simulink library "env2turbLinearize_cl"  (R2020a)
settings: Solver=VariableStepAuto  StartTime=0.0  StopTime=10.0  RelTol=1e-3
undefined symbols (not defined in the file or in its folder): distAmp, distFreq, flwSpd, initializeBussesFromBlock, pertVec, vhcl
libraries: flowcalculation_cl x4, $bdroot x3, eulAng2RotMat_ul x1, alphaBetaLE_ul x1, vrlib x1
settings Model: Creator=mcobb  LastModifiedBy=andre
settings DataIOCC: ReturnWorkspaceOutputs=off
settings DebuggingCC: ArithmeticOperatorsInVariantConditions=warning
settings SFSimCC: CustomCodeUndefinedFunction=UseInterfaceOnly

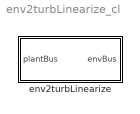
== system env2turbLinearize_cl ==
  env2turbLinearize : Subsystem  LoadFcn=initializeBussesFromBlock(gcb)  InitFcn=initializeBussesFromBlock(gcb)  StartFcn=initializeBussesFromBlock(gcb)
      settings: MinAlgLoopOccurrences=on

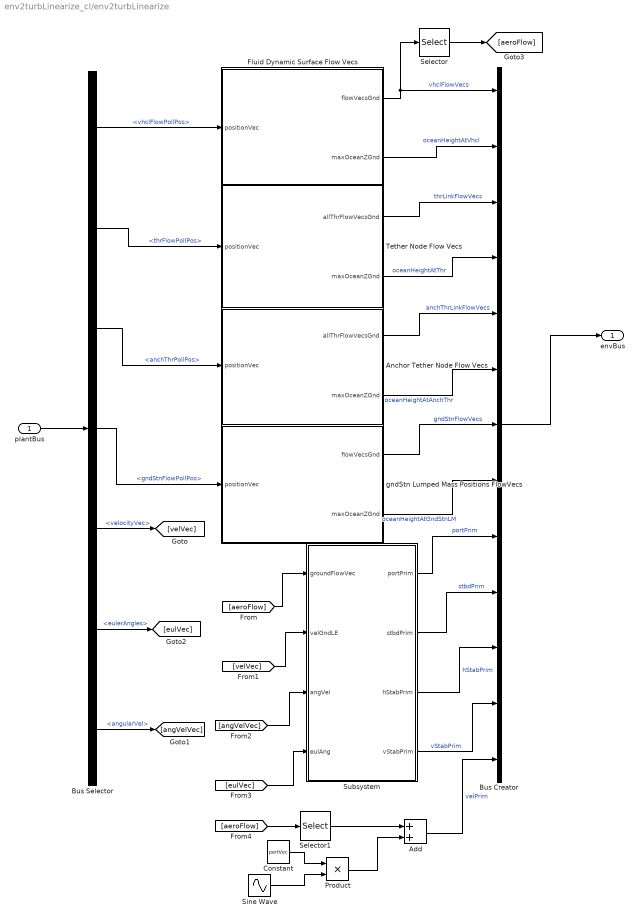
== system env2turbLinearize_cl/env2turbLinearize ==
  plantBus : Inport  OutDataTypeStr=Bus: plantBus
  Add : Sum
  Anchor Tether Node Flow Vecs : Subsystem
  Bus Creator : BusCreator  Inputs=13  OutDataTypeStr=Bus: envBus  NonVirtualBus=on
  Bus Selector : BusSelector  OutputSignals=vhclFlowPollPos,thrFlowPollPos,anchThrPollPos,gndStnFlowPollPos,velocityVec,eulerAngles,angularVel
  Constant : Constant  Value=pertVec
  Fluid Dynamic Surface Flow Vecs : Subsystem
      settings: MinAlgLoopOccurrences=on
  Product : Product
  Selector : Selector  NumberOfDimensions=2  InputPortWidth=[13 3]  IndexOptions=Select all,Index vector (dialog)  Indices=[1 3],[1 2 3 4]  OutputSizes=1,1
  Selector1 : Selector  NumberOfDimensions=2  InputPortWidth=3  IndexOptions=Select all,Index vector (dialog)  Indices=[1 3],1  OutputSizes=1,1
  Sine Wave : Sin  Amplitude=distAmp*flwSpd  Frequency=distFreq*2*pi  SampleTime=[0,1]
  Subsystem : Subsystem  mask{vhcl=vhcl, fluidMomentArms=vhcl.fluidMomentArms.Value}
      mask prompts: vhcl "Vehicle Object"; fluidMomentArms "Fluid Moment Arms"
  Tether Node Flow Vecs : Subsystem
      settings: MinAlgLoopOccurrences=on
  gndStn Lumped Mass Positions FlowVecs : Subsystem
      settings: MinAlgLoopOccurrences=on
  envBus : Outport  OutDataTypeStr=Bus: envBus  VectorParamsAs1DForOutWhenUnconnected=off
  wires:
  Bus Selector/1 -> Fluid Dynamic Surface Flow Vecs/1(positionVec)  "<vhclFlowPollPos>"
  Fluid Dynamic Surface Flow Vecs/1(flowVecsGnd) -> Selector/1, Bus Creator/1  "vhclFlowVecs"
  Bus Creator/1 -> envBus/1
  Bus Selector/3 -> Anchor Tether Node Flow Vecs/1(positionVec)  "<anchThrPollPos>"
  Bus Selector/2 -> Tether Node Flow Vecs/1(positionVec)  "<thrFlowPollPos>"
  plantBus/1 -> Bus Selector/1
  Bus Selector/4 -> gndStn Lumped Mass Positions FlowVecs/1(positionVec)  "<gndStnFlowPollPos>"
  gndStn Lumped Mass Positions FlowVecs/2(maxOceanZGnd) -> Bus Creator/8  "oceanHeightAtGndStnLM"
  Tether Node Flow Vecs/1(allThrFlowVecsGnd) -> Bus Creator/3  "thrLinkFlowVecs"
  Anchor Tether Node Flow Vecs/1(allThrFlowVecsGnd) -> Bus Creator/5  "anchThrLinkFlowVecs"
  gndStn Lumped Mass Positions FlowVecs/1(flowVecsGnd) -> Bus Creator/7  "gndStnFlowVecs"
  Anchor Tether Node Flow Vecs/2(maxOceanZGnd) -> Bus Creator/6  "oceanHeightAtAnchThr"
  Tether Node Flow Vecs/2(maxOceanZGnd) -> Bus Creator/4  "oceanHeightAtThr"
  Fluid Dynamic Surface Flow Vecs/2(maxOceanZGnd) -> Bus Creator/2  "oceanHeightAtVhcl"
  Bus Selector/5 -> [velVec]  "<velocityVec>"
  Bus Selector/7 -> [angVelVec]  "<angularVel>"
  Bus Selector/6 -> [eulVec]  "<eulerAngles>"
  [velVec] -> Subsystem/2(velGndLE)
  Selector/1 -> [aeroFlow]
  [aeroFlow] -> Subsystem/1(groundFlowVec)
  [angVelVec] -> Subsystem/3(angVel)
  [eulVec] -> Subsystem/4(eulAng)
  Subsystem/2(stbdPrim) -> Bus Creator/10  "stbdPrim"
  Subsystem/3(hStabPrim) -> Bus Creator/11  "hStabPrim"
  Subsystem/4(vStabPrim) -> Bus Creator/12  "vStabPrim"
  Subsystem/1(portPrim) -> Bus Creator/9  "portPrim"
  [aeroFlow] -> Selector1/1
  Selector1/1 -> Add/1
  Sine Wave/1 -> Product/2
  Add/1 -> Bus Creator/13  "velPrim"
  Constant/1 -> Product/1
  Product/1 -> Add/2

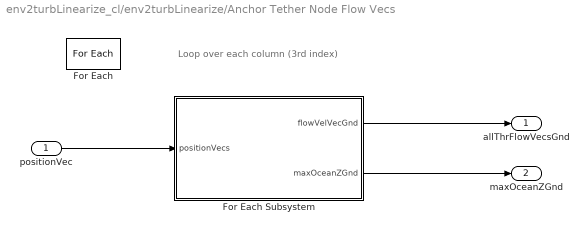
== system env2turbLinearize_cl/env2turbLinearize/Anchor Tether Node Flow Vecs ==
  note: Loop over each column (3rd index)
  positionVec : Inport  Partition=on  PartitionDimension=3  PartitionWidth=1  PartitionOffset=0
  For Each : ForEach  DisableCoverage=on
  For Each Subsystem : Subsystem
      settings: MinAlgLoopOccurrences=on
  allThrFlowVecsGnd : Outport  ConcatenationDimension=3  VectorParamsAs1DForOutWhenUnconnected=off
  maxOceanZGnd : Outport  Port=2  ConcatenationDimension=1  VectorParamsAs1DForOutWhenUnconnected=off
  wires:
  positionVec/1 -> For Each Subsystem/1(positionVecs)
  For Each Subsystem/1(flowVelVecGnd) -> allThrFlowVecsGnd/1
  For Each Subsystem/2(maxOceanZGnd) -> maxOceanZGnd/1

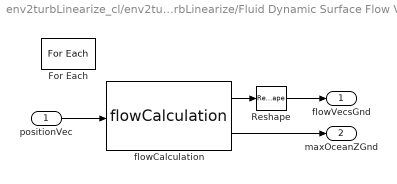
== system env2turbLinearize_cl/env2turbLinearize/Fluid Dynamic Surface Flow Vecs ==
  positionVec : Inport  Partition=on  PartitionDimension=2  PartitionWidth=1  PartitionOffset=0
  For Each : ForEach  DisableCoverage=on
  Reshape : Reshape  OutputDimensionality=Column vector (2-D)
  flowCalculation : flowcalculation_cl/flowCalculation  SystemSampleTime=-1  Latency=0  AutoFrameSizeCalculation=off
  flowVecsGnd : Outport  ConcatenationDimension=2  VectorParamsAs1DForOutWhenUnconnected=off
  maxOceanZGnd : Outport  Port=2  ConcatenationDimension=1  VectorParamsAs1DForOutWhenUnconnected=off
  wires:
  positionVec/1 -> flowCalculation/1
  flowCalculation/1 -> Reshape/1
  Reshape/1 -> flowVecsGnd/1
  flowCalculation/2 -> maxOceanZGnd/1

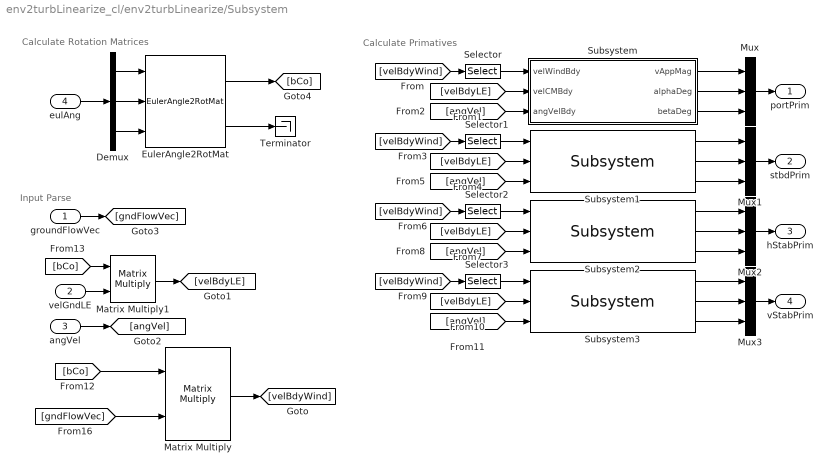
== system env2turbLinearize_cl/env2turbLinearize/Subsystem ==
  note: Calculate Primatives
  note: Calculate Rotation Matrices
  note: Input Parse
  groundFlowVec : Inport
  velGndLE : Inport  Port=2
  angVel : Inport  Port=3
  eulAng : Inport  Port=4
  Demux : Demux  Outputs=3
  EulerAngle2RotMat : eulAng2RotMat_ul/EulerAngle2RotMat  SystemSampleTime=-1  Latency=0  AutoFrameSizeCalculation=off
  Matrix Multiply : Product  Multiplication=Matrix(*)
  Matrix Multiply1 : Product  Multiplication=Matrix(*)
  Mux{,1..3} (4 alike) : Mux  Inputs=3
  Selector : Selector  NumberOfDimensions=2  InputPortWidth=3  IndexOptions=Select all,Index vector (dialog)  Indices=[1 3],1  OutputSizes=1,1
  Selector1 : Selector  NumberOfDimensions=2  InputPortWidth=3  IndexOptions=Select all,Index vector (dialog)  Indices=[1 3],2  OutputSizes=1,1
  Selector2 : Selector  NumberOfDimensions=2  InputPortWidth=3  IndexOptions=Select all,Index vector (dialog)  Indices=[1 3],3  OutputSizes=1,1
  Selector3 : Selector  NumberOfDimensions=2  InputPortWidth=3  IndexOptions=Select all,Index vector (dialog)  Indices=[1 3],4  OutputSizes=1,1
  Subsystem : Subsystem  mask{aSurf=vhcl.portWing, rArm_LE=fluidMomentArms(:,1)}
      mask prompts: aSurf "AeroSurface Object"; rArm_LE "Moment Arm"
  Subsystem1 : $bdroot/environmentManta2RotBandLin/Subsystem/Subsystem  aSurf=vhcl.stbdWing  rArm_LE=fluidMomentArms(:,2)
  Subsystem2 : $bdroot/environmentManta2RotBandLin/Subsystem/Subsystem  aSurf=vhcl.hStab  rArm_LE=fluidMomentArms(:,3)
  Subsystem3 : $bdroot/environmentManta2RotBandLin/Subsystem/Subsystem  aSurf=vhcl.vStab  rArm_LE=fluidMomentArms(:,4)
  Terminator : Terminator
  portPrim : Outport
  stbdPrim : Outport  Port=2
  hStabPrim : Outport  Port=3
  vStabPrim : Outport  Port=4
  wires:
  Demux/3 -> EulerAngle2RotMat/3
  Demux/1 -> EulerAngle2RotMat/1
  Demux/2 -> EulerAngle2RotMat/2
  EulerAngle2RotMat/2 -> Terminator/1
  EulerAngle2RotMat/1 -> [bCo]
  eulAng/1 -> Demux/1
  velGndLE/1 -> Matrix Multiply1/2
  angVel/1 -> [angVel]
  [velBdyWind] -> Selector/1
  [velBdyLE] -> Subsystem/2(velCMBdy)
  [angVel] -> Subsystem/3(angVelBdy)
  Selector/1 -> Subsystem/1(velWindBdy)
  Selector1/1 -> Subsystem1/1
  [angVel] -> Subsystem1/3
  [velBdyWind] -> Selector1/1
  [velBdyLE] -> Subsystem1/2
  Selector2/1 -> Subsystem2/1
  [angVel] -> Subsystem2/3
  [velBdyWind] -> Selector2/1
  [velBdyLE] -> Subsystem2/2
  Selector3/1 -> Subsystem3/1
  [angVel] -> Subsystem3/3
  [velBdyWind] -> Selector3/1
  [velBdyLE] -> Subsystem3/2
  Subsystem/3(betaDeg) -> Mux/3
  Mux/1 -> portPrim/1
  Mux1/1 -> stbdPrim/1
  Mux2/1 -> hStabPrim/1
  Mux3/1 -> vStabPrim/1
  Subsystem1/1 -> Mux1/1
  Subsystem1/3 -> Mux1/3
  Subsystem2/2 -> Mux2/2
  Subsystem2/3 -> Mux2/3
  Subsystem3/1 -> Mux3/1
  Subsystem3/2 -> Mux3/2
  Subsystem3/3 -> Mux3/3
  groundFlowVec/1 -> [gndFlowVec]
  [bCo] -> Matrix Multiply/1
  Matrix Multiply/1 -> [velBdyWind]
  [bCo] -> Matrix Multiply1/1
  Matrix Multiply1/1 -> [velBdyLE]
  [gndFlowVec] -> Matrix Multiply/2
  Subsystem2/1 -> Mux2/1
  Subsystem/1(vAppMag) -> Mux/1
  Subsystem/2(alphaDeg) -> Mux/2
  Subsystem1/2 -> Mux1/2

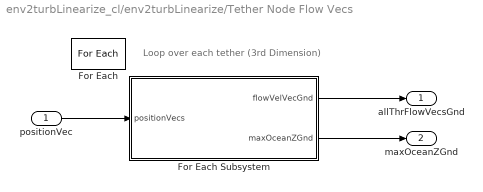
== system env2turbLinearize_cl/env2turbLinearize/Tether Node Flow Vecs ==
  note: Loop over each tether (3rd Dimension)
  positionVec : Inport  Partition=on  PartitionDimension=3  PartitionWidth=1  PartitionOffset=0
  For Each : ForEach  DisableCoverage=on
  For Each Subsystem : Subsystem
      settings: MinAlgLoopOccurrences=on
  allThrFlowVecsGnd : Outport  ConcatenationDimension=3  VectorParamsAs1DForOutWhenUnconnected=off
  maxOceanZGnd : Outport  Port=2  ConcatenationDimension=1  VectorParamsAs1DForOutWhenUnconnected=off
  wires:
  For Each Subsystem/1(flowVelVecGnd) -> allThrFlowVecsGnd/1
  positionVec/1 -> For Each Subsystem/1(positionVecs)
  For Each Subsystem/2(maxOceanZGnd) -> maxOceanZGnd/1

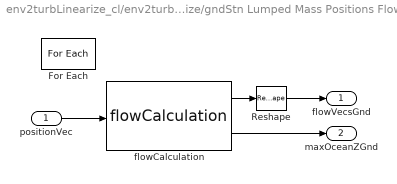
== system env2turbLinearize_cl/env2turbLinearize/gndStn Lumped Mass Positions FlowVecs ==
  positionVec : Inport  Partition=on  PartitionDimension=2  PartitionWidth=1  PartitionOffset=0
  For Each : ForEach  DisableCoverage=on
  Reshape : Reshape  OutputDimensionality=Column vector (2-D)
  flowCalculation : flowcalculation_cl/flowCalculation  SystemSampleTime=-1  Latency=0  AutoFrameSizeCalculation=off
  flowVecsGnd : Outport  ConcatenationDimension=2  VectorParamsAs1DForOutWhenUnconnected=off
  maxOceanZGnd : Outport  Port=2  ConcatenationDimension=1  VectorParamsAs1DForOutWhenUnconnected=off
  wires:
  flowCalculation/2 -> maxOceanZGnd/1
  Reshape/1 -> flowVecsGnd/1
  flowCalculation/1 -> Reshape/1
  positionVec/1 -> flowCalculation/1

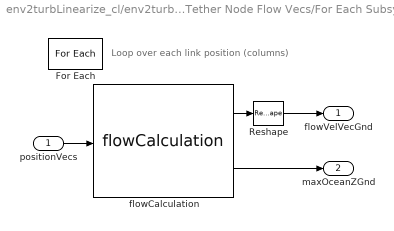
== system env2turbLinearize_cl/env2turbLinearize/Anchor Tether Node Flow Vecs/For Each Subsystem ==
  note: Loop over each link position (columns)
  positionVecs : Inport  Partition=on  PartitionDimension=2  PartitionWidth=1  PartitionOffset=0
  For Each : ForEach  DisableCoverage=on
  Reshape : Reshape  OutputDimensionality=Column vector (2-D)
  flowCalculation : flowcalculation_cl/flowCalculation  SystemSampleTime=-1  Latency=0  AutoFrameSizeCalculation=off
  flowVelVecGnd : Outport  ConcatenationDimension=2  VectorParamsAs1DForOutWhenUnconnected=off
  maxOceanZGnd : Outport  Port=2  ConcatenationDimension=1  VectorParamsAs1DForOutWhenUnconnected=off
  wires:
  flowCalculation/1 -> Reshape/1
  Reshape/1 -> flowVelVecGnd/1
  positionVecs/1 -> flowCalculation/1
  flowCalculation/2 -> maxOceanZGnd/1

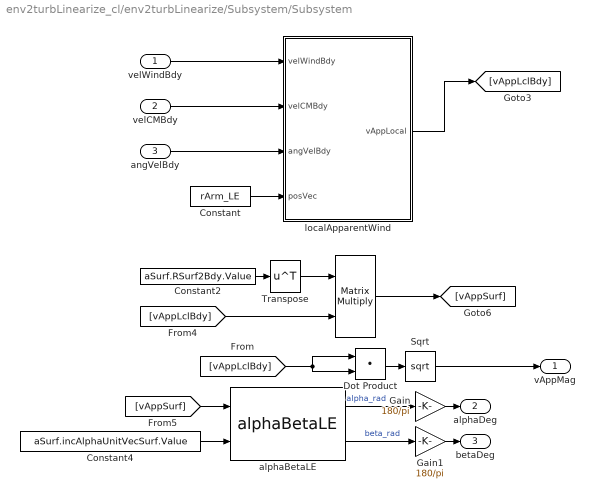
== system env2turbLinearize_cl/env2turbLinearize/Subsystem/Subsystem ==
  velWindBdy : Inport
  velCMBdy : Inport  Port=2
  angVelBdy : Inport  Port=3
  "  " : Product  Multiplication=Matrix(*)
  Constant : Constant  Value=rArm_LE  VectorParams1D=off
  Constant2 : Constant  Value=aSurf.RSurf2Bdy.Value  VectorParams1D=off
  Constant4 : Constant  Value=aSurf.incAlphaUnitVecSurf.Value  VectorParams1D=off
  Dot Product : DotProduct  InputSameDT=on  OutDataTypeStr=Inherit: Inherit via internal rule
  Gain : Gain  Gain=180/pi
  Gain1 : Gain  Gain=180/pi
  Sqrt : Sqrt  SaturateOnIntegerOverflow=on
  Transpose : Math  Operator=transpose  SignedPower=on  SaturateOnIntegerOverflow=on
  alphaBetaLE : alphaBetaLE_ul/alphaBetaLE  SystemSampleTime=-1  Latency=0  AutoFrameSizeCalculation=off
  localApparentWind : Subsystem
  vAppMag : Outport
  alphaDeg : Outport  Port=2
  betaDeg : Outport  Port=3
  wires:
  angVelBdy/1 -> localApparentWind/3(angVelBdy)
  velCMBdy/1 -> localApparentWind/2(velCMBdy)
  Constant/1 -> localApparentWind/4(posVec)
  velWindBdy/1 -> localApparentWind/1(velWindBdy)
  localApparentWind/1(vAppLocal) -> [vAppLclBdy]
  Transpose/1 -> "  "/1
  Constant2/1 -> Transpose/1
  "  "/1 -> [vAppSurf]
  [vAppLclBdy] -> "  "/2
  Constant4/1 -> alphaBetaLE/2
  alphaBetaLE/2 -> Gain1/1  "beta_rad"
  alphaBetaLE/1 -> Gain/1  "alpha_rad"
  [vAppSurf] -> alphaBetaLE/1
  [vAppLclBdy] -> Dot Product/2, Dot Product/1
  Gain/1 -> alphaDeg/1
  Gain1/1 -> betaDeg/1
  Dot Product/1 -> Sqrt/1
  Sqrt/1 -> vAppMag/1

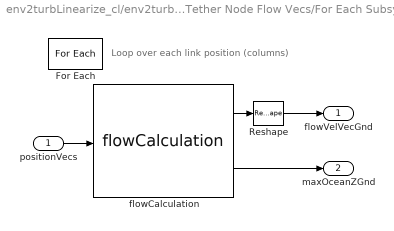
== system env2turbLinearize_cl/env2turbLinearize/Tether Node Flow Vecs/For Each Subsystem ==
  note: Loop over each link position (columns)
  positionVecs : Inport  Partition=on  PartitionDimension=2  PartitionWidth=1  PartitionOffset=0
  For Each : ForEach  DisableCoverage=on
  Reshape : Reshape  OutputDimensionality=Column vector (2-D)
  flowCalculation : flowcalculation_cl/flowCalculation  SystemSampleTime=-1  Latency=0  AutoFrameSizeCalculation=off
  flowVelVecGnd : Outport  ConcatenationDimension=2  VectorParamsAs1DForOutWhenUnconnected=off
  maxOceanZGnd : Outport  Port=2  ConcatenationDimension=1  VectorParamsAs1DForOutWhenUnconnected=off
  wires:
  flowCalculation/1 -> Reshape/1
  Reshape/1 -> flowVelVecGnd/1
  positionVecs/1 -> flowCalculation/1
  flowCalculation/2 -> maxOceanZGnd/1

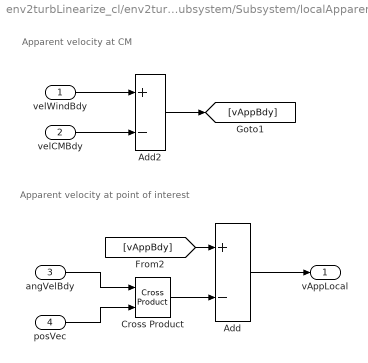
== system env2turbLinearize_cl/env2turbLinearize/Subsystem/Subsystem/localApparentWind ==
  note: Apparent velocity at CM
  note: Apparent velocity at point of interest
  velWindBdy : Inport
  velCMBdy : Inport  Port=2
  angVelBdy : Inport  Port=3
  posVec : Inport  Port=4
  Add : Sum  Inputs=+-
  Add2 : Sum  Inputs=+-
  Cross Product : vrlib/Utilities/Cross Product
  vAppLocal : Outport  VectorParamsAs1DForOutWhenUnconnected=off
  wires:
  angVelBdy/1 -> Cross Product/1
  [vAppBdy] -> Add/1
  Add2/1 -> [vAppBdy]
  velCMBdy/1 -> Add2/2
  velWindBdy/1 -> Add2/1
  Cross Product/1 -> Add/2
  posVec/1 -> Cross Product/2
  Add/1 -> vAppLocal/1
